simulink model "v_YWB_G2s"  (R2016a)
settings: Solver=VariableStepAuto  SolverMode=SingleTasking  StartTime=0.0  StopTime=10  RelTol=1e-3
values from neighbouring files (symbols this model uses):
  dendy = sym2poly(D)    [ac_YWB_G1.m]    (also in step_YWB_G2.m; v_YWB_G1.m; v_YWB_G2.m)
  numdy = sym2poly(N)    [ac_YWB_G1.m]    (also in step_YWB_G2.m; v_YWB_G1.m; v_YWB_G2.m)
libraries: simulink x1
settings Model: Creator=Fish_Schrodinger  LastModifiedBy=Fish_Schrodinger
settings DataIOCC: LimitDataPoints=on  SaveOutput=off  SaveTime=off
settings OptimizationCC: BlockReduction=off  BooleanDataType=off
settings DebuggingCC: SaveWithParameterizedLinksMsg=none  UnderspecifiedInitializationDetection=Classic  MergeDetectMultiDrivingBlocksExec=none  SignalResolutionControl=TryResolveAllWithWarning  AllowSymbolicDim=off
settings HardwareCC: TargetUnknown=on

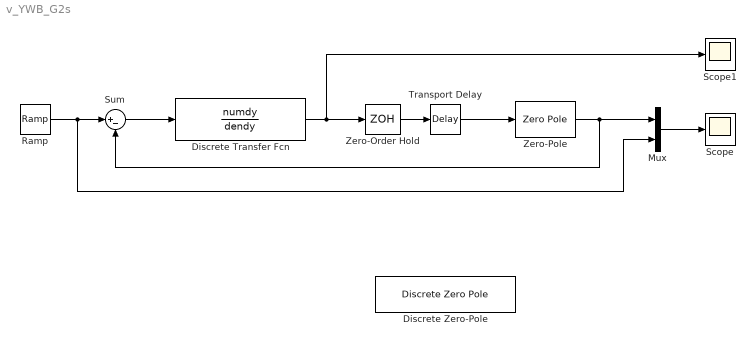
== system v_YWB_G2s ==
  Discrete Transfer Fcn : DiscreteTransferFcn  Numerator=numdy  Denominator=dendy  SampleTime=0.5
  Discrete Zero-Pole : DiscreteZeroPole  Zeros=[0.5 0.3679]  Poles=[1 -0.7183]  Gain=50000/9197/2  SampleTime=0.5
  Mux : Mux  Inputs=2
  Ramp : simulink/Sources/Ramp  slope=1  start=0  X0=0
  Scope : Scope
  Scope1 : Scope
  Sum : Sum  Inputs=|+-
  Transport Delay : TransportDelay
  Zero-Order Hold : ZeroOrderHold  SampleTime=0.5
  Zero-Pole : ZeroPole  Zeros=[]  Poles=[-2]  Gain=[2]
  wires:
  Sum/1 -> Discrete Transfer Fcn/1
  Discrete Transfer Fcn/1 -> Scope1/1, Zero-Order Hold/1
  Zero-Pole/1 -> Mux/1, Sum/2
  Ramp/1 -> Mux/2, Sum/1
  Mux/1 -> Scope/1
  Transport Delay/1 -> Zero-Pole/1
  Zero-Order Hold/1 -> Transport Delay/1
